simulink model "obs_motor_CD_simulink"  (R2020a)
settings: Solver=VariableStepAuto  StartTime=0.0  StopTime=10.0  RelTol=1e-3
values from neighbouring files (symbols this model uses):
  A = [-3, 2, 0 ... (first row only)    [AsesoriaP3.m]    (also in Circ_Doble_Malla_ODE_plot.m = [0, 1/C2; -1/(R1*C1*R2), -(C2*R1+C2*R2+R1*C1)/(C1*C2*R1*R2)]; ControlThis_P1.m = [-1,-3,0; Controlador_Retro_plot.m = [0, 0, 1, 0; Engranes_ODE_plot.m = [0, 1; -K./(Jm2 + Jm1.*(n2./n1)^2), -B/(Jm2 + Jm1.*(n2./n1)^)
  B = [2, 0 ... (first row only)    [AsesoriaP3.m]    (also in Circ_Doble_Malla_ODE_plot.m = [0; 1/(C1*R1*R2)]; ControlThis_P1.m = [2,4,2; Controlador_Retro_plot.m = [0; Engranes_ODE_plot.m = [0; -1/(n1.*Jm2/2 + n2.*Jm1./n1)])
  C = [0, 3, 0]    [AsesoriaP3.m]    (also in Circ_Doble_Malla_ODE_plot.m = [1 0]; ControlThis_P1.m = [3,2,0; Controlador_Retro_plot.m = [1, 0, 0, 0]; Engranes_ODE_plot.m = [1, 0])
  L = -Ho*inv(Mo)*[0;1]    [Ex3_ej2.m]    (also in Exam_sys_plot.m = 0.002; LQR_motor_cd_plot.m = 0.005; Tarea_31.m = -Ho*inv(Mo)*[0;0;1]; motor_cd_plot.m = 0.005)
settings Model: Creator=micro microndas  LastModifiedBy=micro microndas

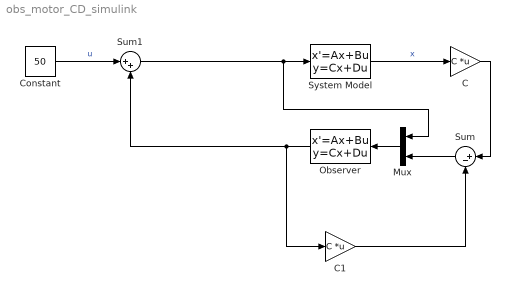
== system obs_motor_CD_simulink ==
  C : Gain  Gain=C  Multiplication=Matrix(K*u)
  C1 : Gain  Gain=C  Multiplication=Matrix(K*u)
  Constant : Constant  Value=50
  Mux : Mux  Inputs=2
  Observer : StateSpace  A=A  B=[B, -L]  C=eye(2)  D=[0, 0;0, 0]  InitialCondition=0
  Sum : Sum  Inputs=|+-
  Sum1 : Sum  Inputs=|++
  System Model : StateSpace  A=A  B=B  C=eye(2)  D=[0;0];  InitialCondition=[5, 4]
  wires:
  System Model/1 -> C/1  "x"
  C/1 -> Sum/1
  C1/1 -> Sum/2
  Observer/1 -> Sum1/2, C1/1
  Constant/1 -> Sum1/1  "u"
  Sum1/1 -> Mux/1, System Model/1
  Mux/1 -> Observer/1
  Sum/1 -> Mux/2
